simulink model "d5_b_2_model"  (R2025a)
settings: Solver=VariableStepAuto  StartTime=0.0  StopTime=10.0  RelTol=1e-3
values from neighbouring files (symbols this model uses):
  Ts = 0.001    [d5_b_1.m]    (also in d5_b_2.m)
  w = 1    [d5_a_2.m]    (also in d5_b_2.m)
settings Model: Creator=Korisnik  LastModifiedBy=Korisnik

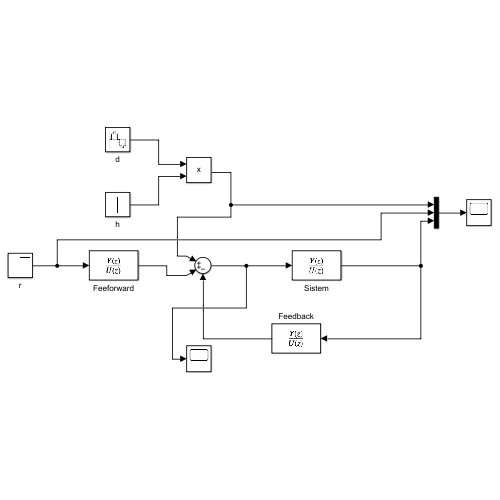
[thumbnail: Simulink's stored preview of the top-level diagram]
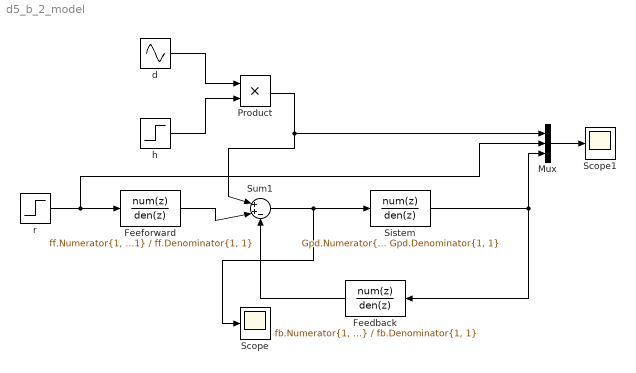
== system d5_b_2_model ==
  Feedback : DiscreteTransferFcn  Numerator=fb.Numerator{1, 1}  Denominator=fb.Denominator{1, 1}
  Feeforward : DiscreteTransferFcn  Numerator=ff.Numerator{1, 1}  Denominator=ff.Denominator{1, 1}
  Mux : Mux  Inputs=3
  Product : Product
  Scope : Scope
      settings: ActiveDisplayYMinimum=-1.8705394645531102  ActiveDisplayYMaximum=2.2773582878214507
  Scope1 : Scope
      settings: ActiveDisplayYMinimum=-0.64749  ActiveDisplayYMaximum=5.82738
  Sistem : DiscreteTransferFcn  Numerator=Gpd.Numerator{1, 1}  Denominator=Gpd.Denominator{1, 1}
  Sum1 : Sum  Inputs=|++-
  d : Sin  Frequency=w  SampleTime=Ts
  h : Step  Time=3  SampleTime=Ts
  r : Step  Time=0  After=5  SampleTime=Ts
  wires:
  r/1 -> Mux/2, Feeforward/1
  Sum1/1 -> Scope/1, Sistem/1
  Sistem/1 -> Mux/3, Feedback/1
  h/1 -> Product/2
  d/1 -> Product/1
  Product/1 -> Mux/1, Sum1/1
  Feeforward/1 -> Sum1/2
  Feedback/1 -> Sum1/3
  Mux/1 -> Scope1/1
